simulink model "P_HIL_Inverse_Motor_model"  (R2019b)
settings: Solver=VariableStepAuto  StartTime=0.0  StopTime=10.0  RelTol=1e-3
values from neighbouring files (symbols this model uses):
  kszi0 = (sqrt(2)*(Un_RMS/sqrt(3)))/(2*pi*fn)    [PHIL_dummy_motor.m]
  Ld = L    [PHIL_dummy_motor.m]
  Lq = L    [PHIL_dummy_motor.m]
  pp = 1    [PHIL_dummy_motor.m]
  Rs = (X_Rr * Zn)    [PHIL_dummy_motor.m]
  Theta = (Pn*T_start)/(omega_n^2)    (= 0.0911890652781)    [PHIL_dummy_motor.m]
libraries: coordinate_transformations x4
settings Model: Creator=kissd  LastModifiedBy=kissd

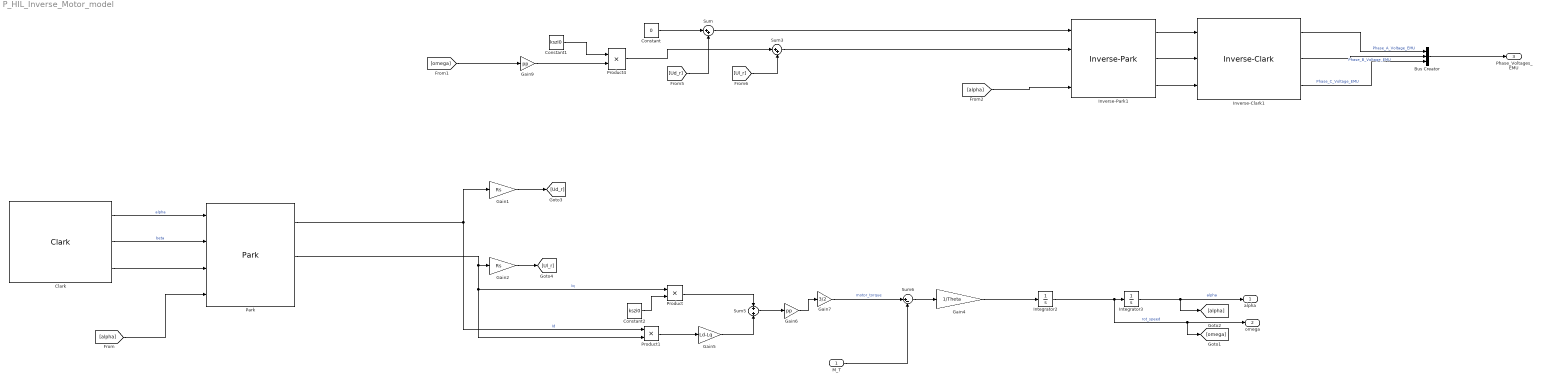
== system P_HIL_Inverse_Motor_model ==
  M_T : Inport
  Bus Creator : BusCreator  Inputs=3
  Clark : coordinate_transformations/Clark  SystemSampleTime=-1  Latency=0  AutoFrameSizeCalculation=off
  Constant : Constant  Value=0
  Constant1 : Constant  Value=kszi0
  Constant2 : Constant  Value=kszi0
  Gain1 : Gain  Gain=Rs
  Gain2 : Gain  Gain=Rs
  Gain4 : Gain  Gain=1/Theta
  Gain5 : Gain  Gain=Ld-Lq
  Gain6 : Gain  Gain=pp
  Gain7 : Gain  Gain=3/2
  Gain9 : Gain  Gain=pp
  Integrator2 : Integrator
  Integrator3 : Integrator
  Inverse-Clark1 : coordinate_transformations/Inverse-Clark  SystemSampleTime=-1  Latency=0  AutoFrameSizeCalculation=off
  Inverse-Park1 : coordinate_transformations/Inverse-Park  SystemSampleTime=-1  Latency=0  AutoFrameSizeCalculation=off
  Park : coordinate_transformations/Park  SystemSampleTime=-1  Latency=0  AutoFrameSizeCalculation=off
  Product : Product
  Product1 : Product
  Product4 : Product
  Sum : Sum  Inputs=|++
  Sum3 : Sum  Inputs=|++
  Sum5 : Sum  Inputs=+|+
  Sum6 : Sum  Inputs=|+-
  alpha : Outport
  omega : Outport  Port=2
  Phase_Voltages_EMU : Outport  Port=3
  wires:
  Constant1/1 -> Product4/1
  Sum6/1 -> Gain4/1
  Constant/1 -> Sum/1
  Gain4/1 -> Integrator2/1
  Product4/1 -> Sum3/1
  [omega] -> Gain9/1
  Product1/1 -> Gain5/1
  [alpha] -> Inverse-Park1/4
  [Ul_r] -> Sum3/2
  Gain9/1 -> Product4/2
  [Ud_r] -> Sum/2
  Sum3/1 -> Inverse-Park1/2
  Sum/1 -> Inverse-Park1/1
  Inverse-Clark1/3 -> Bus Creator/3  "Phase_C_Voltage_EMU"
  Inverse-Park1/1 -> Inverse-Clark1/1
  Inverse-Clark1/1 -> Bus Creator/1  "Phase_A_Voltage_EMU"
  Inverse-Clark1/2 -> Bus Creator/2  "Phase_B_Voltage_EMU"
  Park/2 -> Product1/2, Product/1, Gain2/1  "Iq"
  Product/1 -> Sum5/1
  Sum5/1 -> Gain6/1
  Constant2/1 -> Product/2
  Gain6/1 -> Gain7/1
  Park/1 -> Gain1/1, Product1/1  "Id"
  Bus Creator/1 -> Phase_Voltages_EMU/1
  Integrator2/1 -> Integrator3/1, [omega], omega/1  "rot_speed"
  Integrator3/1 -> alpha/1, [alpha]  "alpha"
  Gain5/1 -> Sum5/2
  Inverse-Park1/2 -> Inverse-Clark1/2
  M_T/1 -> Sum6/2
  Gain7/1 -> Sum6/1  "motor_torque"
  Inverse-Park1/3 -> Inverse-Clark1/3
  Gain2/1 -> [Ul_r]
  Gain1/1 -> [Ud_r]
  Clark/1 -> Park/1  "alpha"
  Clark/2 -> Park/2  "beta"
  Clark/3 -> Park/3
  [alpha] -> Park/4
